simulink model "Automatisierung_subsystem"  (R2016b)
settings: Solver=ode1  StartTime=0.0  StopTime=100  FixedStep=0.001  RelTol=1e-3
PostLoadFcn:
  | , if any(exist('dsrtsu_mdlpostloadfcn', 'file') == [2, 3, 6]), try dsrtsu_mdlpostloadfcn('Execute', bdroot); catch fprintf('Error in PostLoadFcn (dsrtsu_mdlpostloadfcn) for model "%s":\n %s\n', bdroot, lasterr); end, end,
undefined symbols (not defined in the file or in its folder): param
PreSaveFcn:
  | , if any(exist('dsmpb_private', 'file') == [2, 3, 6]), try, dsmpb_private('dsmpb_mdlclblib', 'PreSave', bdroot); catch, disp(lasterr); end, end,
CloseFcn:
  | , if any(exist('dsmpb_private', 'file') == [2, 3, 6]), try, dsmpb_private('dsmpb_mdlclblib', 'Close', bdroot); catch, disp(lasterr); end, end,
settings Model: DSRTSU_INTERNAL_RTI_VER=490  DSRTSU_INTERNAL_RTI_TYPE=rti1202  DSRTSU_INTERNAL_RTIFPGA=80  DSMPB_DATASERVER_ModelPortLibVersion1=8  DSMPB_DATASERVER_DataServerVersion1=6  DSMPB_DATASERVER_DataServerStreamVersion1=3  ParamWorkspaceSource=ReferencedWorkspace  Creator=verladebruecke  LastModifiedBy=Fritz
settings OptimizationCC: BlockReduction=off  OptimizeBlockIOStorage=off  BufferReuse=off  GlobalBufferReuse=off  ExpressionFolding=off  LocalBlockOutputs=off
settings HardwareCC: ProdBitPerPointer=32  ProdBitPerSizeT=32  ProdBitPerPtrDiffT=32  ProdLargestAtomicInteger=Integer  ProdEndianess=BigEndian  ProdWordSize=32  ProdHWDeviceType=Custom Processor->Custom  TargetIntDivRoundTo=Zero  TargetEndianess=BigEndian  TargetHWDeviceType=Custom Processor->Custom
settings RTWCC: SystemTargetFile=rti1202.tlc  MakeCommand=make_rti  TemplateMakefile=rti1202.tmf  Description=dSPACE DS1202 Hardware Platform
settings STFCustomTargetCC: ParMdlRefBuildCompliant=on  GRTInterface=off  SystemTargetFile=rti1202.tlc
settings GRTTargetCC: TargetLangStandard=C89/C90 (ANSI)  CompOptLevelCompliant=off  ConcurrentExecutionCompliant=off  CombineOutputUpdateFcns=off  MatFileLogging=off  CPPClassGenCompliant=off  UseToolchainInfoCompliant=off
settings ConfigComp: CovMetricSettings=dswe

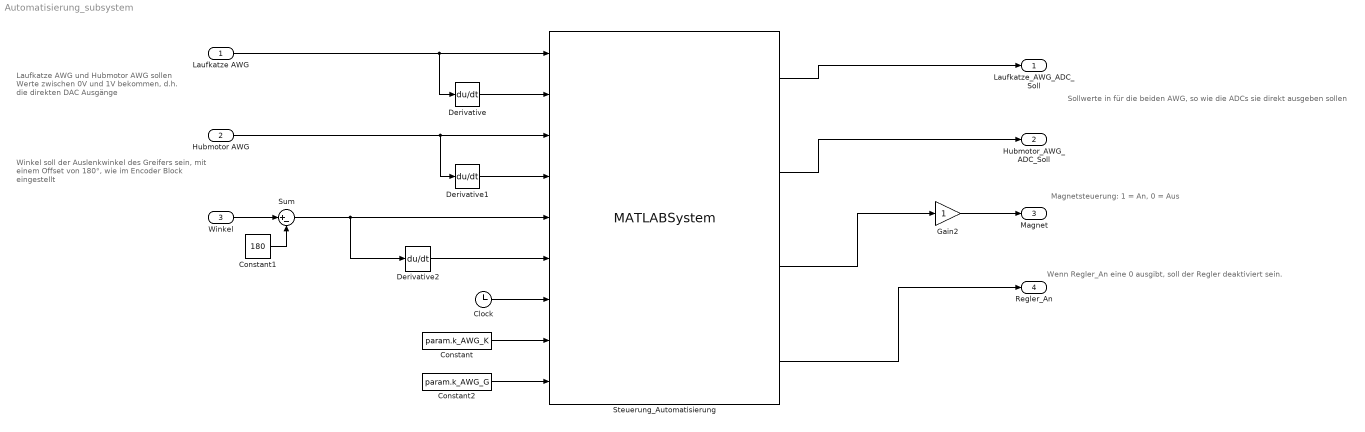
== system Automatisierung_subsystem ==
  note: Magnetsteuerung: 1 = An, 0 = Aus
  note: Sollwerte in für die beiden AWG, so wie die ADCs sie direkt ausgeben sollen
  note: Wenn Regler_An eine 0 ausgibt, soll der Regler deaktiviert sein.
  note: Winkel soll der Auslenkwinkel des Greifers sein,
      | mit einem Offset von 180°, wie im
      | Encoder Block eingestellt
  note: Laufkatze AWG und Hubmotor AWG sollen
      | Werte zwischen 0V und 1V bekommen,
      | d.h. die direkten DAC Ausgänge
  Laufkatze AWG : Inport  OutMin=0  OutMax=1  OutDataTypeStr=double  PortDimensions=1
  Hubmotor AWG : Inport  Port=2  OutMin=0  OutMax=1  OutDataTypeStr=double  PortDimensions=1
  Winkel : Inport  Port=3  OutMin=0  OutMax=360  OutDataTypeStr=double  PortDimensions=1
  Clock : Clock
  Constant : Constant  Value=param.k_AWG_K
  Constant1 : Constant  Value=180
  Constant2 : Constant  Value=param.k_AWG_G
  Derivative : Derivative
  Derivative1 : Derivative
  Derivative2 : Derivative
  Gain2 : Gain
  Steuerung_Automatisierung : MATLABSystem  System=Steuerung_Automatisierung  box_sequence=box_sequence  start_time=start_time  add_midpoints=true  SimulateUsing=Code generation
      mask Type: Steuerung_Automatisierung
      mask Display:
      | disp('Steuerung_Automatisierung');
      | port_label('input',1,'horiz_value');
      | port_label('input',2,'horiz_speed');
      | port_label('input',3,'vert_value');
      | port_label('input',4,'vert_speed');
      | port_label('input',5,'angle');
      | port_label('input',6,'angle_speed');
      | port_label('input',7,'Clock');
      | port_label('input',8,'k_AWG_K');
      | port_label('input',9,'k_AWG_G');
      | port_label('output',1,'horiz_setpoint');
      | port_label('output',2,'vert_setpoint');
      | port_label('output',3,'magnet_on');
      | port_label('output',4,'control_enable');
  Sum : Sum  Inputs=|+-
  Laufkatze_AWG_ADC_Soll : Outport  SignalName=Laufkatze_AWG_ADC_Soll
  Hubmotor_AWG_ADC_Soll : Outport  Port=2  SignalName=Hubmotor_AWG_ADC_Soll
  Magnet : Outport  Port=3  SignalName=Magnet
  Regler_An : Outport  Port=4  SignalName=Regler_An
  wires:
  Derivative/1 -> Steuerung_Automatisierung/2
  Derivative1/1 -> Steuerung_Automatisierung/4
  Derivative2/1 -> Steuerung_Automatisierung/6
  Laufkatze AWG/1 -> Derivative/1, Steuerung_Automatisierung/1
  Hubmotor AWG/1 -> Derivative1/1, Steuerung_Automatisierung/3
  Constant1/1 -> Sum/2
  Winkel/1 -> Sum/1
  Sum/1 -> Steuerung_Automatisierung/5, Derivative2/1
  Steuerung_Automatisierung/3 -> Gain2/1
  Steuerung_Automatisierung/4 -> Regler_An/1
  Steuerung_Automatisierung/2 -> Hubmotor_AWG_ADC_Soll/1
  Steuerung_Automatisierung/1 -> Laufkatze_AWG_ADC_Soll/1
  Gain2/1 -> Magnet/1
  Clock/1 -> Steuerung_Automatisierung/7
  Constant/1 -> Steuerung_Automatisierung/8
  Constant2/1 -> Steuerung_Automatisierung/9
